simulink model "TST_DYN_ORB_V2"  (R2020a)
settings: Solver=VariableStepAuto  StartTime=0.0  StopTime=10000  RelTol=1e-3
undefined symbols (not defined in the file): DYN_SC_par
libraries: DYN_ATT x1, DYN_EPHEM x1, DYN_GRAV x1, DYN_TIME x1, DYN_TRA x1
settings Model: Creator=WilTravis  LastModifiedBy=m_mam
settings DataIOCC: ReturnWorkspaceOutputs=off
settings DebuggingCC: ArithmeticOperatorsInVariantConditions=warning
settings SFSimCC: SimUseLocalCustomCode=off  CustomCodeUndefinedFunction=UseInterfaceOnly
settings RTWCC: RTWUseLocalCustomCode=off

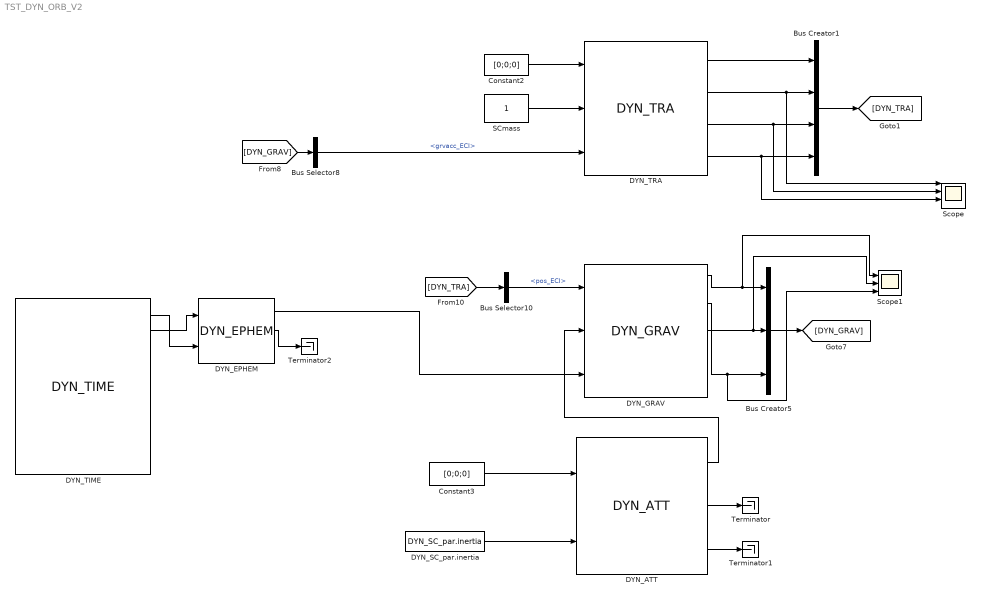
== system TST_DYN_ORB_V2 ==
  Bus Creator1 : BusCreator  Inputs=4
  Bus Creator5 : BusCreator  Inputs=3
  Bus Selector10 : BusSelector  OutputSignals=pos_ECI
  Bus Selector8 : BusSelector  OutputSignals=grvacc_ECI
  Constant2 : Constant  Value=[0;0;0]
  Constant3 : Constant  Value=[0;0;0]
  DYN_ATT : DYN_ATT/DYN_ATT  SystemSampleTime=-1  Latency=0  AutoFrameSizeCalculation=off
  DYN_EPHEM : DYN_EPHEM/DYN_EPHEM  SystemSampleTime=-1  Latency=0  AutoFrameSizeCalculation=off
  DYN_GRAV : DYN_GRAV/DYN_GRAV  SystemSampleTime=-1  Latency=0  AutoFrameSizeCalculation=off
  "DYN_SC_par.inertia " : Constant  Value=DYN_SC_par.inertia
  DYN_TIME : DYN_TIME/DYN_TIME  SystemSampleTime=-1  Latency=0  AutoFrameSizeCalculation=off
  DYN_TRA : DYN_TRA/DYN_TRA  SystemSampleTime=-1  Latency=0  AutoFrameSizeCalculation=off
  SCmass : Constant
  Scope : Scope  NumInputPorts=4
  Scope1 : Scope  NumInputPorts=3
  Terminator : Terminator
  Terminator1 : Terminator
  Terminator2 : Terminator
  wires:
  [DYN_GRAV] -> Bus Selector8/1
  DYN_GRAV/2 -> Scope1/2, Bus Creator5/2
  Constant2/1 -> DYN_TRA/1
  Bus Selector8/1 -> DYN_TRA/3  "<grvacc_ECI>"
  [DYN_TRA] -> Bus Selector10/1
  DYN_TRA/3 -> Scope/2, Bus Creator1/3
  SCmass/1 -> DYN_TRA/2
  DYN_GRAV/3 -> Scope1/3, Bus Creator5/3
  Bus Selector10/1 -> DYN_GRAV/1  "<pos_ECI>"
  Bus Creator5/1 -> [DYN_GRAV]
  DYN_TRA/2 -> Scope/1, Bus Creator1/2
  DYN_TRA/4 -> Scope/3, Bus Creator1/4
  DYN_TRA/1 -> Bus Creator1/1
  DYN_GRAV/1 -> Scope1/1, Bus Creator5/1
  Bus Creator1/1 -> [DYN_TRA]
  "DYN_SC_par.inertia "/1 -> DYN_ATT/2
  Constant3/1 -> DYN_ATT/1
  DYN_ATT/1 -> DYN_GRAV/2
  DYN_ATT/2 -> Terminator/1
  DYN_ATT/3 -> Terminator1/1
  DYN_EPHEM/1 -> DYN_GRAV/3
  DYN_EPHEM/2 -> Terminator2/1
  DYN_TIME/2 -> DYN_EPHEM/1
  DYN_TIME/1 -> DYN_EPHEM/2
